simulink model "Kalman_Upward"  (R2022b)
settings: Solver=ode1  StartTime=0.0  StopTime=40  FixedStep=0.0005  RelTol=1e-3  EnableMultiTasking=on
PostLoadFcn:
  | qc_set_target_type(getConfigSet(bdroot, 'QUARC Default Target Configuration'));
undefined symbols (not defined in the file): Ad, Bd, Cd, Dd, Discrete, HIL, ic, K_pp, qc_get_step_size, Time, ts
libraries: quarc_library x7, simulink_extras x2, dspsrcs4 x2, ctrlSharedLib x1
settings Model: SimulationMode=external  ExtModeTrigDuration=1000000  Creator=CFulford  LastModifiedBy=Utente
settings SolverCC: AlgebraicLoopSolver=TrustRegion  PositivePriorityOrder=on  AutoInsertRateTranBlk=on
settings DataIOCC: LimitDataPoints=on  SaveFormat=Array  SignalLoggingSaveFormat=ModelDataLogs  ReturnWorkspaceOutputs=off
settings OptimizationCC: ExpressionDepthLimit=2147483647  InitFltsAndDblsToZero=on
settings DebuggingCC: SaveWithParameterizedLinksMsg=none  UnderspecifiedInitializationDetection=Classic  MergeDetectMultiDrivingBlocksExec=none  SolverPrmCheckMsg=warning  MultiTaskDSMMsg=warning  MultiTaskCondExecSysMsg=none  FcnCallInpInsideContextMsg=warning  UnconnectedInputMsg=warning  UnconnectedOutputMsg=warning  UnconnectedLineMsg=warning  StateNameClashWarn=warning  SFUnexpectedBacktrackingDiag=warning  SFNoUnconditionalDefaultTransitionDiag=warning  SFExecutionAtInitializationDiag=none  SFMachineParentedDataDiag=warning  ArithmeticOperatorsInVariantConditions=warning
settings ModelReferenceCC: EnableRefExpFcnMdlSchedulingChecks=on  PropagateSignalLabelsOutOfModel=off
settings SFSimCC: SimUseLocalCustomCode=off  CustomCodeUndefinedFunction=UseInterfaceOnly
settings RTWCC: Description=QUARC Win64 Target Using Toolchain  SystemTargetFile=quarc_win64.tlc  TemplateMakefile=quarc_default_tmf  RTWUseLocalCustomCode=off  Toolchain=QUARC win64 | nmake (64-bit Windows)  BuildConfiguration=Faster Runs
settings CodeAppCC: StateflowObjectComments=on
settings STFCustomTargetCC: ConcurrentExecutionCompliant=on  GRTInterface=on  UseToolchainInfoCompliant=on  SystemTargetFile=quarc_win64.tlc
settings GRTTargetCC: TargetLangStandard=C89/C90 (ANSI)  ParMdlRefBuildCompliant=off  CompOptLevelCompliant=off  CombineOutputUpdateFcns=off  MatFileLogging=off  CPPClassGenCompliant=off  GRTInterface=on  ExtMode=on  ExtModeMexFile=quarc_comm
settings ConfigComp: CovMetricSettings=dw  CovSaveCumulativeToWorkspaceVar=on  CovSaveSingleToWorkspaceVar=on  CovExternalEMLEnable=off  CovSFcnEnable=off

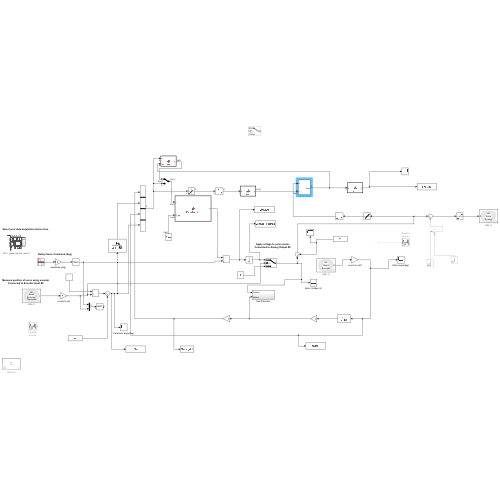
[thumbnail: Simulink's stored preview of the top-level diagram]
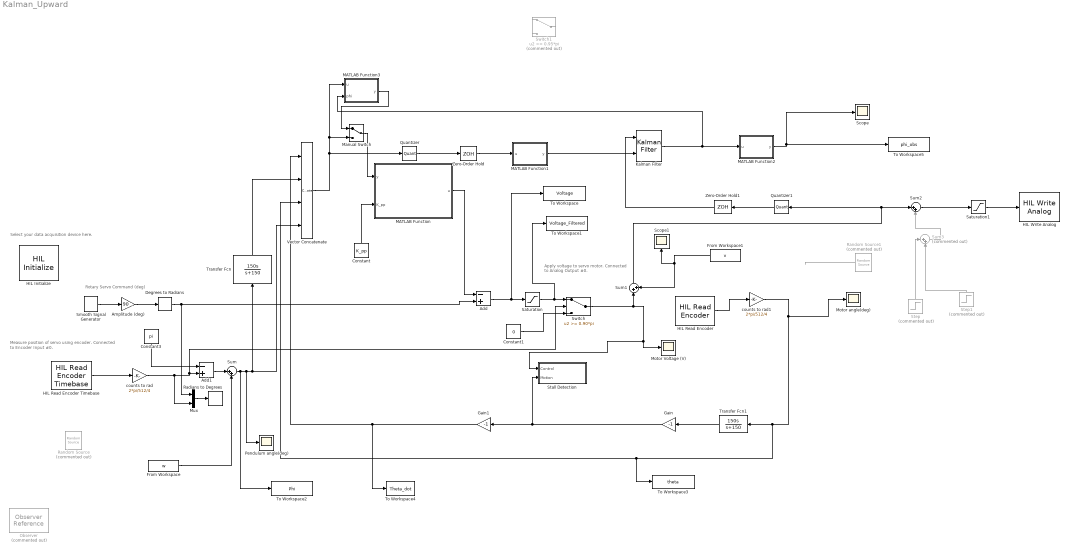
== system Kalman_Upward ==
  note: Rotary Servo Command (deg)
  note: Apply voltage to servo motor.
      | Connected to Analog Output #0.
  note: Measure position of servo using encoder.
      | Connected to Encoder Input #0.
  note: Select your data acquisition device here.
  Add : Sum  Inputs=-+
  Add1 : Sum  Inputs=-+
  Amplitude (deg) : Gain  Gain=90
  Constant : Constant  Value=K_pp  VectorParams1D=off
  Constant1 : Constant  Value=0
  Constant3 : Constant  Value=pi
  Degrees to Radians : simulink_extras/Transformations/Degrees to Radians
  From Workspace : FromWorkspace  VariableName=w
  From Workspace1 : FromWorkspace  VariableName=v
  Gain : Gain  Gain=-1
  Gain1 : Gain  Gain=-1
  HIL Initialize : quarc_library/Data Acquisition/Generic/Configuration/HIL Initialize  Priority=-99  object_name=HIL-1  board_type=qube_servo2_usb  board_number=0  board_options=""  exclusive=off  active=off  hardware_clocks=[0]  clock_modes=[]  initial_clock_frequencies=[]  set_clock_params_at_start=off  set_clock_params_at_switch_in=off  set_clock_frequencies_at_start=off  set_clock_frequencies_at_switch_in=off  analog_input_channels=[0]  analog_input_configurations=[]  analog_input_maximums=3  analog_input_minimums=-3  set_analog_input_params_at_start=off  set_analog_input_params_at_switch_in=off  analog_output_channels=[0]  analog_output_maximums=15  analog_output_minimums=-15  initial_analog_outputs=[0]  final_analog_outputs=[0]  watchdog_analog_outputs=0  set_analog_output_params_at_start=off  set_analog_output_params_at_switch_in=off  set_analog_outputs_at_start=on  set_analog_outputs_at_switch_in=off  set_analog_outputs_at_terminate=on  set_analog_outputs_at_switch_out=off  set_analog_outputs_on_watchdog=on  digital_input_channels=[]  digital_output_channels=[0]  digital_output_configuration=[]  initial_digital_outputs=[1]  final_digital_outputs=[0]  watchdog_digital_outputs=[0]  set_digital_output_params_at_start=off  set_digital_output_params_at_switch_in=off  set_digital_outputs_at_start=on  set_digital_outputs_at_switch_in=off  set_digital_outputs_at_terminate=on  set_digital_outputs_at_switch_out=off  set_digital_outputs_on_watchdog=on  encoder_channels=[0:1]  quadrature=[4]  encoder_filter_frequency=[]  initial_encoder_counts=[0]  set_encoder_params_at_start=off  set_encoder_params_at_switch_in=off  set_encoder_counts_at_start=on  set_encoder_counts_at_switch_in=off  pwm_channels=[]  pwm_modes=[]  pwm_frequency=[]  pwm_configuration=[]  pwm_alignment=[]  pwm_polarity=[]  pwm_leading_deadband=[]  pwm_trailing_deadband=[]  initial_pwm_outputs=[]  final_pwm_outputs=[]  watchdog_pwm_outputs=[]  set_pwm_params_at_start=off  set_pwm_params_at_switch_in=off  set_pwm_outputs_at_start=off  set_pwm_outputs_at_switch_in=off  set_pwm_outputs_at_terminate=off  set_pwm_outputs_at_switch_out=off  set_pwm_outputs_on_watchdog=off  other_output_channels=[11000:11002]  initial_other_outputs=[0 1 0]  final_other_outputs=[1 0 0]  watchdog_other_outputs=[0 0 1]  set_other_outputs_at_start=on  set_other_outputs_at_switch_in=off  set_other_outputs_at_terminate=on  set_other_outputs_at_switch_out=off  set_other_outputs_on_watchdog=on
  HIL Read Encoder : quarc_library/Data Acquisition/Generic/Immediate I//O/HIL Read Encoder  object_name=HIL-1  channels=[0]  sample_time=qc_get_step_size  active=on  vector_output=off  data_type_mode=Inherit via back propagation  data_type=double
  HIL Read Encoder Timebase : quarc_library/Data Acquisition/Generic/Timebases/HIL Read Encoder Timebase  object_name=HIL-1  clock=0  channels=1  active=on  vector_output=off  data_type_mode=Inherit via back propagation  data_type=double  overflow_mode=Error on overflow  samples_in_buffer=max(ceil(1/qc_get_step_size), 1)
  HIL Write Analog : quarc_library/Data Acquisition/Generic/Immediate I//O/HIL Write Analog  object_name=HIL-1  channels=0  sample_time=-1  active=off  vector_input=off
  Kalman Filter : ctrlSharedLib/Kalman Filter  TimeDomain=Discrete-Time  UseCurrentEstimator=on  ModelSource=Individual A, B, C, D matrices  ModelSourceVariable=ss(0.95,1,1,0,1)  A=Ad  B=Bd  C=Cd  D=Dd  NumberOfStates=1  NumberOfInputs=1  NumberOfOutputs=1  InitialEstimateSource=Dialog  X0=ic  P0=10  UseK=off  UseGH=off  NumberOfProcessNoiseInputs=1  G=1  TimeInvariantG=on  H=0  TimeInvariantH=on  Q=0.01  TimeInvariantQ=on  R=0.01  TimeInvariantR=on  N=0  TimeInvariantN=on  AddInputPort=on  AddEnablePort=off  OutputEstimatedY=off  OutputP=off  Ts=-1
  MATLAB Function : MATLAB Function  TreatAsAtomicUnit=on
  MATLAB Function1 : MATLAB Function  TreatAsAtomicUnit=on
  MATLAB Function2 : MATLAB Function  TreatAsAtomicUnit=on
  MATLAB Function3 : MATLAB Function  TreatAsAtomicUnit=on
  Manual Switch : ManualSwitch
  Motor Voltage (V) : Scope
  Motor angle(deg) : Scope
  Mux : Mux  Inputs=2
  Observer : ObserverReference  Commented=on  ObserverModelName=Kalman_Upward_Observer1
  Pendulum angle(deg) : Scope
  Quantizer : Quantizer  QuantizationInterval=ts
  Quantizer1 : Quantizer  QuantizationInterval=ts
  Radians to Degrees : simulink_extras/Transformations/Radians to Degrees
  Random Source : dspsrcs4/Random Source  Commented=on  SrcType=Gaussian  NormMethod=Ziggurat  CltLength=12  MinVal=0  MaxVal=1  MeanVal=0  VarVal=0.001  RepMode=Repeatable  rawSeed=1  IsInherit=off  SampMode=Discrete  SampTime=ts*10  SampFrame=1  DataType=Double  OutComplex=Real  OutputFrames=off
  Random Source1 : dspsrcs4/Random Source  Commented=on  SrcType=Gaussian  NormMethod=Ziggurat  CltLength=12  MinVal=0  MaxVal=1  MeanVal=0  VarVal=0.001  RepMode=Repeatable  rawSeed=1  IsInherit=off  SampMode=Discrete  SampTime=ts*10  SampFrame=1  DataType=Double  OutComplex=Real  OutputFrames=off
  Saturation : Saturate  UpperLimit=5  LowerLimit=-5
  Saturation1 : Saturate  UpperLimit=5  LowerLimit=-5
  Scope : Scope
  Scope1 : Scope
  Smooth Signal Generator : quarc_library/Sources/Signals/Smooth Signal Generator  signal_type=Sine  source=Internal (dialog parameters)  amplitude=0  frequency=1  initial_phase=0  sample_time=qc_get_step_size  output_cos=off
      settings: SourceProductName=QUARC Targets
  Stall Detection : Subsystem
  Step : Step  Commented=on  Time=5  SampleTime=0
  Step1 : Step  Commented=on  Time=6  Before=1  After=0  SampleTime=0
  Sum : Sum  Inputs=|++
  Sum1 : Sum  Inputs=|++
  Sum2 : Sum  Inputs=|++
  Sum3 : Sum  Commented=on  Inputs=|++
  Switch : Switch  Threshold=0.90*pi  SaturateOnIntegerOverflow=off  InputSameDT=off
  Switch1 : Switch  Commented=on  Threshold=0.95*pi  SaturateOnIntegerOverflow=off  InputSameDT=off
  To Workspace : ToWorkspace  VariableName=Voltage  SaveFormat=Structure With Time  SampleTime=-1
  To Workspace1 : ToWorkspace  VariableName=Voltage_Filtered  SaveFormat=Structure With Time  SampleTime=-1
  To Workspace2 : ToWorkspace  VariableName=Phi  SaveFormat=Structure With Time  SampleTime=-1
      settings: Save2DSignal=2-D array (concatenate along first dimension)
  To Workspace3 : ToWorkspace  VariableName=theta  SaveFormat=Structure With Time  SampleTime=-1
  To Workspace4 : ToWorkspace  VariableName=Theta_dot  SaveFormat=Structure With Time  SampleTime=-1
  To Workspace5 : ToWorkspace  VariableName=phi_obs  SaveFormat=Structure With Time  SampleTime=-1
  Transfer Fcn : TransferFcn  Numerator=[150 0]  Denominator=[1 150]
  Transfer Fcn1 : TransferFcn  Numerator=[150 0]  Denominator=[1 150]
  Vector Concatenate : Concatenate  NumInputs=4
  Zero-Order Hold : ZeroOrderHold  SampleTime=ts
  Zero-Order Hold1 : ZeroOrderHold  SampleTime=ts
  counts to rad : Gain  Gain=2*pi/512/4
  counts to rad1 : Gain  Gain=2*pi/512/4
  wires:
  counts to rad/1 -> Switch/2, Add1/2, Mux/2
  Mux/1 -> Radians to Degrees/1
  HIL Read Encoder Timebase/1 -> counts to rad/1
  HIL Read Encoder/1 -> counts to rad1/1
  Saturation/1 -> To Workspace1/1, Switch/1
  Transfer Fcn/1 -> Vector Concatenate/2
  Transfer Fcn1/1 -> Gain/1
  Add/1 -> To Workspace/1, Saturation/1
  MATLAB Function/1(u) -> Add/1
  Degrees to Radians/1 -> Add/2, Mux/1
  Gain1/1 -> To Workspace4/1, Vector Concatenate/1
  Gain/1 -> Gain1/1, Stall Detection/2(Motion)
  Constant/1 -> MATLAB Function/2(K_pp)
  counts to rad1/1 -> Motor angle(deg)/1, Transfer Fcn1/1, To Workspace3/1, Vector Concatenate/3
  Amplitude (deg)/1 -> Degrees to Radians/1
  Smooth Signal Generator/1 -> Amplitude (deg)/1
  Constant3/1 -> Add1/1
  Sum1/1 -> Sum2/1, Quantizer1/1
  Switch/1 -> Stall Detection/1(Control), Motor Voltage (V)/1, Sum1/1
  Vector Concatenate/1 -> Quantizer/1, MATLAB Function3/1(u), Manual Switch/2
  Constant1/1 -> Switch/3
  MATLAB Function2/1(y) -> Scope/1, To Workspace5/1
  Kalman Filter/1 -> MATLAB Function3/2(phi), MATLAB Function2/1(u)
  MATLAB Function1/1(y) -> Kalman Filter/2
  Quantizer/1 -> Zero-Order Hold/1
  Quantizer1/1 -> Zero-Order Hold1/1
  Zero-Order Hold/1 -> MATLAB Function1/1(u)
  Zero-Order Hold1/1 -> Kalman Filter/1
  Add1/1 -> Sum/1
  Sum/1 -> To Workspace2/1, Pendulum angle(deg)/1, Vector Concatenate/4, Transfer Fcn/1
  MATLAB Function3/1(y) -> Manual Switch/1
  Manual Switch/1 -> MATLAB Function/1(y)
  Random Source1/1 -> ?
  Sum2/1 -> Saturation1/1
  Saturation1/1 -> HIL Write Analog/1
  Step/1 -> Sum3/1
  Step1/1 -> Sum3/2
  Sum3/1 -> Sum2/2
  From Workspace/1 -> Sum/2
  From Workspace1/1 -> Scope1/1, Sum1/2

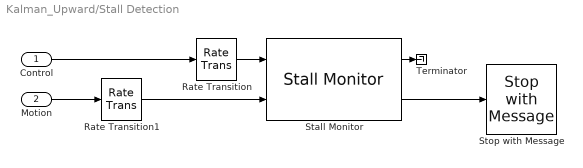
== system Kalman_Upward/Stall Detection ==
  Control : Inport
  Motion : Inport  Port=2
  Rate Transition : RateTransition
  Rate Transition1 : RateTransition
  Stall Monitor : quarc_library/Discrete/Stall Monitor  control_threshold=5  motion_threshold=0.3  duration_s=0.05
      settings: SourceProductName=QUARC Targets
  Stop with Message : quarc_library/Sinks/Error Handling/Stop with Message  message_type=Fixed error message  message_icon=Error  message=Stall Detected! Please ensure that the DC motor is free to move and is functioning properly
  Terminator : Terminator
  wires:
  Control/1 -> Rate Transition/1
  Motion/1 -> Rate Transition1/1
  Stall Monitor/2 -> Stop with Message/1
  Stall Monitor/1 -> Terminator/1
  Rate Transition/1 -> Stall Monitor/1
  Rate Transition1/1 -> Stall Monitor/2

== matlab function Kalman_Upward/MATLAB Function1 ==
  data: u input; y output
function y = fcn(u)
y = [u(1) u(2) u(4)]';

== matlab function Kalman_Upward/MATLAB Function ==
  data: y input; u output; K_pp input

function u = Multiplication(y,K_pp)
%K_pp = [-1.2343   -4.2371   -1.0000  -48.2020];

u = K_pp*y;

end

== matlab function Kalman_Upward/MATLAB Function2 ==
  data: u input; y output
function y = fcn(u)
y = u(3);

== matlab function Kalman_Upward/MATLAB Function3 ==
  data: u input; y output; phi input
function y = fcn(u,phi)
u(4) = phi(3);
u(2) = phi(2);
u(1) = phi(1);
y = u;
